simulink model "tut02"  (R2024b)
settings: Solver=VariableStepAuto  StartTime=0.0  StopTime=10.0  RelTol=1e-3
libraries: NSA_DEVS_LOGISTICS x3, NSA_DEVS_SINKS x3, NSA_DEVS_SOURCES x1
settings Model: Creator=peter  LastModifiedBy=peter

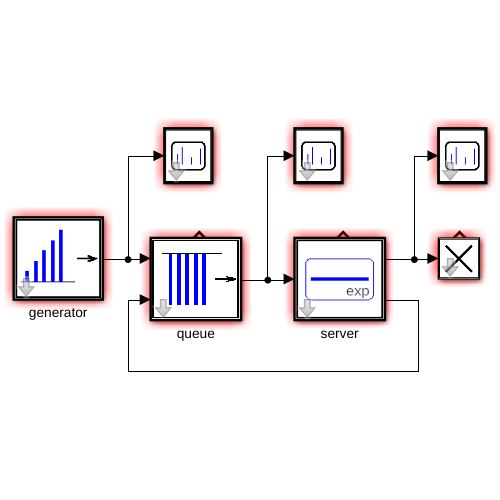
[thumbnail: Simulink's stored preview of the top-level diagram]
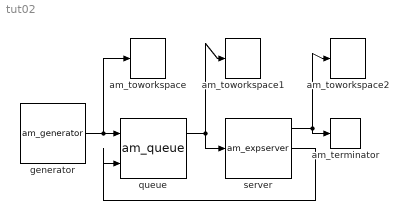
== system tut02 ==
  am_terminator : NSA_DEVS_LOGISTICS/am_terminator  tau=[0,1]  debug=0
      settings: SourceProductName=Logistics
  am_toworkspace : NSA_DEVS_SINKS/am_toworkspace  varname="\"gen\""  t0=0  format="\"vector\""  tau=[0,5]  debug=0
      settings: SourceProductName=Sinks
  am_toworkspace1 : NSA_DEVS_SINKS/am_toworkspace  varname="\"srvIn\""  t0=0  format="\"vector\""  tau=[0,5]  debug=0
      settings: SourceProductName=Sinks
  am_toworkspace2 : NSA_DEVS_SINKS/am_toworkspace  varname="\"srvOut\""  t0=0  format="\"vector\""  tau=[0,5]  debug=0
      settings: SourceProductName=Sinks
  generator : NSA_DEVS_SOURCES/am_generator  tG=1  n0=1  nG=inf  tD=[0,2]  debug=0
      settings: SourceProductName=Sources
  queue : NSA_DEVS_LOGISTICS/am_queue  tD=[0,2]  tau=[0,1]  debug=0
      settings: SourceProductName=Logistics
  server : NSA_DEVS_LOGISTICS/am_expserver  tS=1.0  useSeed=true  seed=3  tau=[0,1]  debug=0
      settings: SourceProductName=Logistics
  wires:
  server/1 -> am_toworkspace2/1, am_terminator/1
  server/2 -> queue/2
  generator/1 -> am_toworkspace/1, queue/1
  queue/1 -> server/1, am_toworkspace1/1
